simulink model "pstCtrl_testV1"  (R2015a)
settings: Solver=ode45  StartTime=0.0  StopTime=inf  FixedStep=0.05  RelTol=1e-3
values from neighbouring files (symbols this model uses):
  g = 9.81    [PosCntrl_Params.m]
  k_f = m*g/omega_h^2    (= 1.18520816327e-09)    [PosCntrl_Params.m]
  Kdz = 0.4    [PosCntrl_Params.m]
  Kpz = 1.2    [PosCntrl_Params.m]
  m = 0.037    [PosCntrl_Params.m]
  omega_h = 17500    [PosCntrl_Params.m]
  pitch_lb = -40*pi/180    (= -0.698131700798)    [PosCntrl_Params.m]
  pitch_ub = 40*pi/180    (= 0.698131700798)    [PosCntrl_Params.m]
  roll_lb = -40*pi/180    (= -0.698131700798)    [PosCntrl_Params.m]
  roll_ub = 40*pi/180    (= 0.698131700798)    [PosCntrl_Params.m]
  yaw_lb = -pi    (= -3.14159265359)    [PosCntrl_Params.m]
  yaw_ub = pi    (= 3.14159265359)    [PosCntrl_Params.m]
undefined symbols (not defined in the file or in its folder): Kdxx, Kdyy, Kpxy, Kpyx
libraries: aerolibconvert2 x4, CrazyFlie_lib x2, realtime_pacer_lib x2, robotlib x2
settings Model: Creator=rshu  LastModifiedBy=rshu

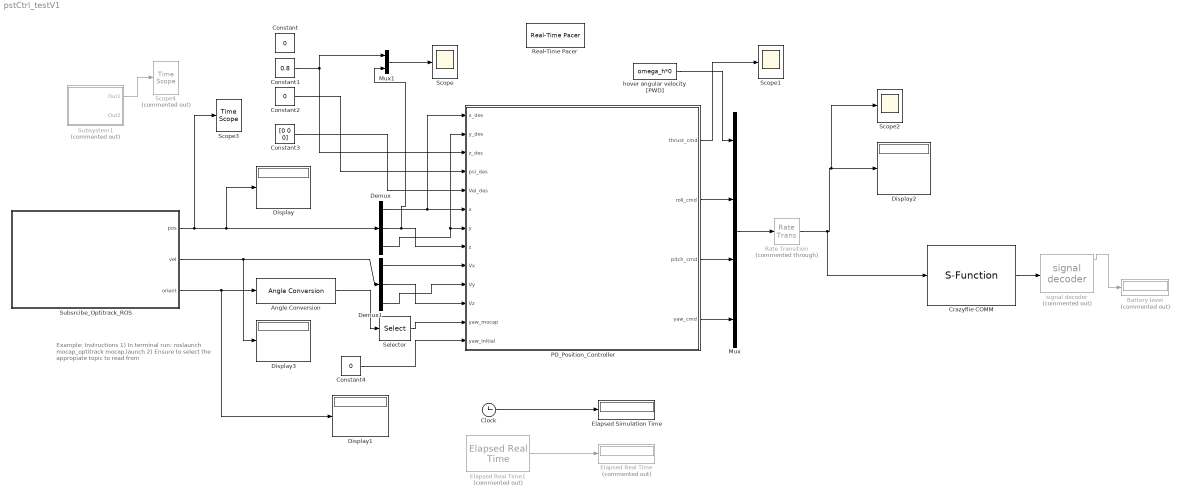
== system pstCtrl_testV1 ==
  note: Example:
      |
      | Instructions
      | 1) In terminal run:
      | roslaunch mocap_optitrack mocap.launch
      | 2) Ensure to select the appropiate topic to read from
  Angle Conversion : aerolibconvert2/Angle Conversion  IU=deg  OU=rad
  Battery level : Display  Commented=on
      settings: Decimation=2
  Clock : Clock
  Constant : Constant  Value=0
  Constant1 : Constant  Value=0.8
  Constant2 : Constant  Value=0
  Constant3 : Constant  Value=[0 0 0]
  Constant4 : Constant  Value=0
  Crazyflie COMM : CrazyFlie_lib/S-Function
  Demux : Demux  Outputs=3
  Demux1 : Demux  Outputs=3
  Display{,1..3} (4 alike) : Display
  Elapsed Real Time : Display  Commented=on
      settings: Decimation=2
  Elapsed Real Time1 : realtime_pacer_lib/Elapsed Real Time  Commented=on
  Elapsed Simulation Time : Display
      settings: Decimation=2
  Mux : Mux
  Mux1 : Mux  Inputs=2
  PD_Position_Controller : Subsystem
  Rate Transition : RateTransition  RequirementInfo="{}  %GIDa_a2c92fb4_87a0_42dd_9129_8c73b2091979"  Commented=through  OutPortSampleTime=sample_time
  Real-Time Pacer : realtime_pacer_lib/Real-Time Pacer  simTimePerRealTime=1
  Scope : Scope
      settings: YMin=0.65  YMax=1
  Scope1 : Scope
      settings: YMin=50468.8  YMax=55781.2
  Scope2 : Scope
      settings: YMin=50468.8  YMax=55781.2  SaveName=ScopeData6
  Scope3 : TimeScope
  Scope4 : TimeScope  Commented=on
  Selector : Selector  InputPortWidth=3  Indices=[2]
  Subsrcibe_Optitrack_ROS : Subsystem
      mask Display:
      | image('prime41-optitrack.png');
      | color('cyan')
      | port_label('output',1,'pos [vector]');
      | port_label('output',2,'vel [vector]');
      | port_label('output',3,'orient [euler]');
  Subsystem1 : Subsystem  Commented=on
  hover angular velocity [PWD] : Constant  Value=omega_h*0
  signal decoder : CrazyFlie_lib/signal decoder  Commented=on
  wires:
  Subsrcibe_Optitrack_ROS/1(pos) -> Demux/1, Display/1, Scope3/1
  Subsrcibe_Optitrack_ROS/2(vel) -> Display3/1, Demux1/1
  Demux/1 -> PD_Position_Controller/1(x_des), PD_Position_Controller/6(x)
  Demux1/1 -> PD_Position_Controller/9(Vx)
  Selector/1 -> PD_Position_Controller/12(yaw_mocap)
  Constant2/1 -> PD_Position_Controller/4(psi_des)
  Constant3/1 -> PD_Position_Controller/5(Vel_des)
  Constant4/1 -> PD_Position_Controller/13(yaw_initial)
  PD_Position_Controller/3(pitch_cmd) -> Mux/3
  PD_Position_Controller/2(roll_cmd) -> Mux/2
  PD_Position_Controller/4(yaw_cmd) -> Mux/4
  Mux/1 -> Rate Transition/1
  Demux/2 -> Mux1/2, PD_Position_Controller/8(z)
  Demux/3 -> PD_Position_Controller/2(y_des), PD_Position_Controller/7(y)
  Demux1/2 -> PD_Position_Controller/11(Vz)
  Demux1/3 -> PD_Position_Controller/10(Vy)
  Constant1/1 -> PD_Position_Controller/3(z_des), Mux1/1
  Subsrcibe_Optitrack_ROS/3(orient) -> Display1/1, Angle Conversion/1
  Angle Conversion/1 -> Selector/1
  Mux1/1 -> Scope/1
  Clock/1 -> Elapsed Simulation Time/1
  Elapsed Real Time1/1 -> Elapsed Real Time/1
  Crazyflie COMM/1 -> signal decoder/1
  signal decoder/1 -> Battery level/1
  PD_Position_Controller/1(thrust_cmd) -> Scope1/1
  hover angular velocity [PWD]/1 -> Mux/1
  Rate Transition/1 -> Crazyflie COMM/1, Scope2/1, Display2/1
  Subsystem1/1(Out1) -> Scope4/1

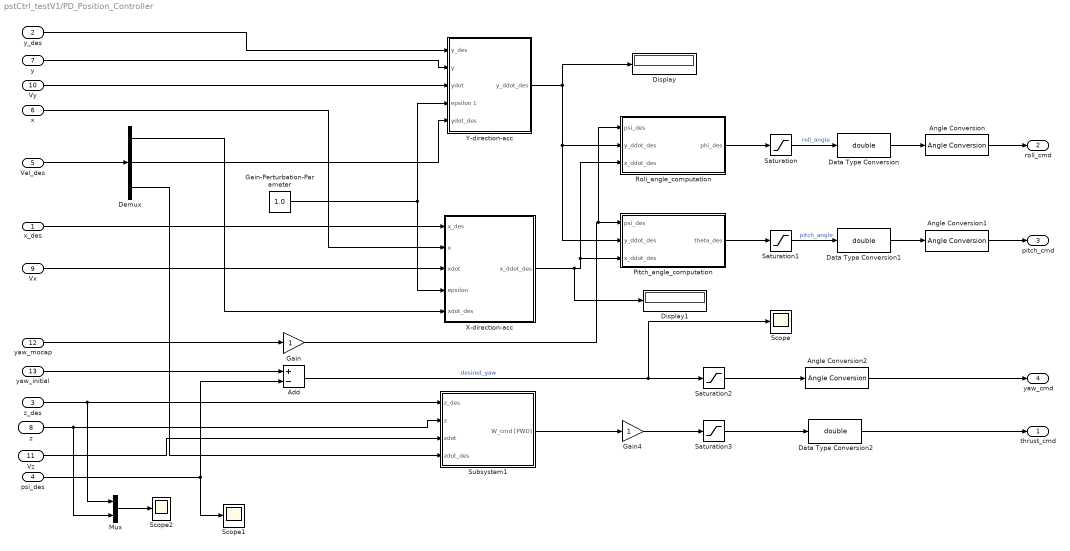
== system pstCtrl_testV1/PD_Position_Controller ==
  x_des : Inport
  y_des : Inport  Port=2
  z_des : Inport  Port=3
  psi_des : Inport  Port=4
  Vel_des : Inport  Port=5
  x : Inport  Port=6
  y : Inport  Port=7
  z : Inport  Port=8
  Vx : Inport  Port=9
  Vy : Inport  Port=10
  Vz : Inport  Port=11
  yaw_mocap : Inport  Port=12
  yaw_initial : Inport  Port=13
  Add : Sum  Inputs=+-
  Angle Conversion : aerolibconvert2/Angle Conversion  IU=rad  OU=deg
  Angle Conversion1 : aerolibconvert2/Angle Conversion  IU=rad  OU=deg
  Angle Conversion2 : aerolibconvert2/Angle Conversion  IU=rad  OU=deg
  Data Type Conversion : DataTypeConversion  OutDataTypeStr=double
  Data Type Conversion1 : DataTypeConversion  OutDataTypeStr=double
  Data Type Conversion2 : DataTypeConversion  OutDataTypeStr=double
  Demux : Demux  Outputs=3
  Display : Display
  Display1 : Display
  Gain : Gain
  Gain-Perturbation-Parameter : Constant  Value=1.0
  Gain4 : Gain
  Mux : Mux  Inputs=2
  Pitch_angle_computation : Subsystem
  Roll_angle_computation : Subsystem
  Saturation : Saturate  UpperLimit=roll_ub  LowerLimit=roll_lb
  Saturation1 : Saturate  UpperLimit=pitch_ub  LowerLimit=pitch_lb
  Saturation2 : Saturate  UpperLimit=yaw_ub  LowerLimit=yaw_lb
  Saturation3 : Saturate  UpperLimit=6e4  LowerLimit=omega_h
  Scope : Scope
      settings: YMin=-1  YMax=1.5  SaveName=ScopeData35
  Scope1 : Scope
      settings: SaveName=ScopeData37
  Scope2 : Scope
      settings: YMin=0.65  YMax=1  SaveName=ScopeData5
  Subsystem1 : Subsystem
  X-direction-acc : Subsystem
  Y-direction-acc : Subsystem
  thrust_cmd : Outport
  roll_cmd : Outport  Port=2
  pitch_cmd : Outport  Port=3
  yaw_cmd : Outport  Port=4
  wires:
  Gain-Perturbation-Parameter/1 -> X-direction-acc/4("epsilon "), Y-direction-acc/4(epsilon 1)
  Roll_angle_computation/1("phi_des ") -> Saturation/1
  Pitch_angle_computation/1("theta_des ") -> Saturation1/1
  X-direction-acc/1(x_ddot_des) -> Display1/1, Roll_angle_computation/3("x_ddot_des "), Pitch_angle_computation/3("x_ddot_des ")
  Y-direction-acc/1(y_ddot_des) -> Roll_angle_computation/2(y_ddot_des), Pitch_angle_computation/2(y_ddot_des), Display/1
  Vy/1 -> Y-direction-acc/3("ydot ")
  Vz/1 -> Subsystem1/3("zdot ")
  y/1 -> Y-direction-acc/2(y)
  Vx/1 -> X-direction-acc/3("xdot ")
  x/1 -> X-direction-acc/2(x)
  Saturation1/1 -> Data Type Conversion1/1  "pitch_angle"
  Saturation/1 -> Data Type Conversion/1  "roll_angle"
  yaw_initial/1 -> Add/1
  Add/1 -> Scope/1, Saturation2/1  "desired_yaw"
  Saturation2/1 -> Angle Conversion2/1
  psi_des/1 -> Scope1/1, Add/2
  z_des/1 -> Mux/1, Subsystem1/1(z_des)
  yaw_mocap/1 -> Gain/1
  Gain/1 -> Roll_angle_computation/1("psi_des "), Pitch_angle_computation/1("psi_des ")
  Gain4/1 -> Saturation3/1
  x_des/1 -> X-direction-acc/1(x_des)
  y_des/1 -> Y-direction-acc/1(y_des)
  Vel_des/1 -> Demux/1
  Demux/2 -> Y-direction-acc/5(ydot_des)
  Demux/1 -> X-direction-acc/5(xdot_des)
  Demux/3 -> Subsystem1/4(zdot_des)
  Data Type Conversion1/1 -> Angle Conversion1/1
  Data Type Conversion2/1 -> thrust_cmd/1
  Data Type Conversion/1 -> Angle Conversion/1
  Angle Conversion/1 -> roll_cmd/1
  Angle Conversion1/1 -> pitch_cmd/1
  Angle Conversion2/1 -> yaw_cmd/1
  Saturation3/1 -> Data Type Conversion2/1
  Subsystem1/1(W_cmd [PWD]) -> Gain4/1
  Mux/1 -> Scope2/1
  z/1 -> Mux/2, Subsystem1/2(z)

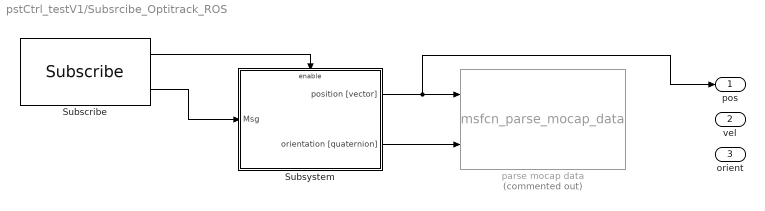
== system pstCtrl_testV1/Subsrcibe_Optitrack_ROS ==
  Subscribe : robotlib/Subscribe  SourceLibraryInfo=This block requires Robotics System Toolbox  topicSource=Select from ROS network  topic=/CF/pose  messageType=geometry_msgs/PoseStamped  sampleTime=-1  messageQueueLength=1
  Subsystem : Subsystem
  parse mocap data : M-S-Function  Commented=on  FunctionName=msfcn_parse_mocap_data
      mask Display:
      | port_label('input', 1, 'pos')
      | port_label('input', 2, 'ornt')
      | 
      | port_label('output', 1, 'pos')
      | port_label('output', 2, 'vel')
      | port_label('output', 3, 'ornt [Euler]')
  pos : Outport
  vel : Outport  Port=2
  orient : Outport  Port=3
  wires:
  Subsystem/1(position [vector]) -> pos/1, parse mocap data/1
  Subscribe/2 -> Subsystem/1(Msg)
  Subscribe/1 -> Subsystem/Enable
  Subsystem/2(orientation [quaternion]) -> parse mocap data/2

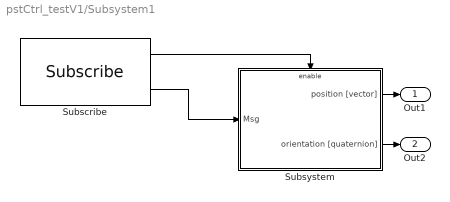
== system pstCtrl_testV1/Subsystem1 ==
  Subscribe : robotlib/Subscribe  SourceLibraryInfo=This block requires Robotics System Toolbox  topicSource=Select from ROS network  topic=/turtle2/pose  messageType=turtlesim/Pose  sampleTime=-1  messageQueueLength=1
  Subsystem : Subsystem
  Out1 : Outport
  Out2 : Outport  Port=2
  wires:
  Subscribe/2 -> Subsystem/1(Msg)
  Subscribe/1 -> Subsystem/Enable
  Subsystem/1(position [vector]) -> Out1/1
  Subsystem/2(orientation [quaternion]) -> Out2/1

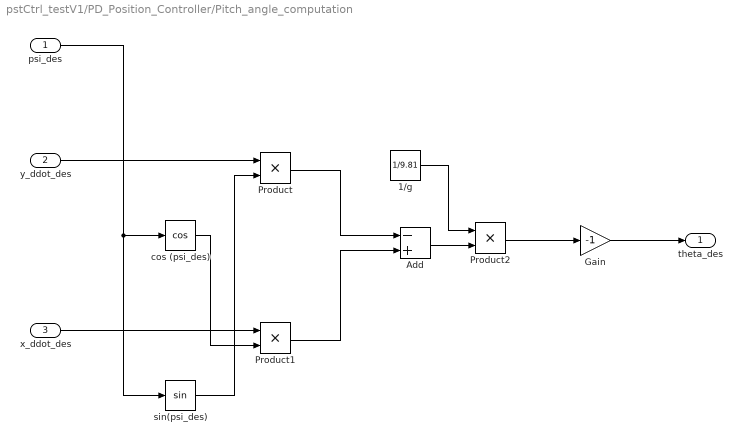
== system pstCtrl_testV1/PD_Position_Controller/Pitch_angle_computation ==
  "psi_des " : Inport
  y_ddot_des : Inport  Port=2
  "x_ddot_des " : Inport  Port=3
  "1/g " : Constant  Value=1/9.81
  Add : Sum  Inputs=-+
  Gain : Gain  Gain=-1
  Product : Product
  Product1 : Product
  Product2 : Product
  cos (psi_des) : Trigonometry  Operator=cos
  sin(psi_des) : Trigonometry
  "theta_des " : Outport
  wires:
  "psi_des "/1 -> cos (psi_des)/1, sin(psi_des)/1
  y_ddot_des/1 -> Product/1
  "x_ddot_des "/1 -> Product1/1
  Product/1 -> Add/1
  Product1/1 -> Add/2
  Add/1 -> Product2/2
  "1/g "/1 -> Product2/1
  Product2/1 -> Gain/1
  Gain/1 -> "theta_des "/1
  cos (psi_des)/1 -> Product1/2
  sin(psi_des)/1 -> Product/2

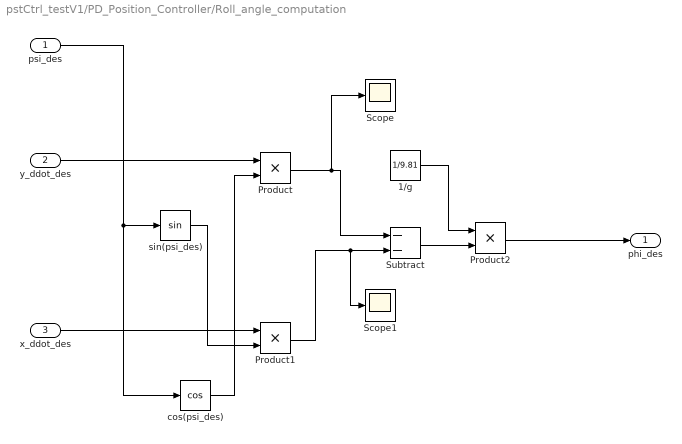
== system pstCtrl_testV1/PD_Position_Controller/Roll_angle_computation ==
  "psi_des " : Inport
  y_ddot_des : Inport  Port=2
  "x_ddot_des " : Inport  Port=3
  "1/g " : Constant  Value=1/9.81
  Product : Product
  Product1 : Product
  Product2 : Product
  Scope : Scope
      settings: TimeRange=30  YMin=-30  YMax=20  SaveName=ScopeData28
  Scope1 : Scope
      settings: TimeRange=30  YMin=-61.5  YMax=-61.3  SaveName=ScopeData30
  Subtract : Sum  Inputs=--
  cos(psi_des) : Trigonometry  Operator=cos
  sin(psi_des) : Trigonometry
  "phi_des " : Outport
  wires:
  "psi_des "/1 -> cos(psi_des)/1, sin(psi_des)/1
  y_ddot_des/1 -> Product/1
  "x_ddot_des "/1 -> Product1/1
  Product/1 -> Scope/1, Subtract/1
  Product1/1 -> Scope1/1, Subtract/2
  Subtract/1 -> Product2/2
  "1/g "/1 -> Product2/1
  Product2/1 -> "phi_des "/1
  sin(psi_des)/1 -> Product1/2
  cos(psi_des)/1 -> Product/2

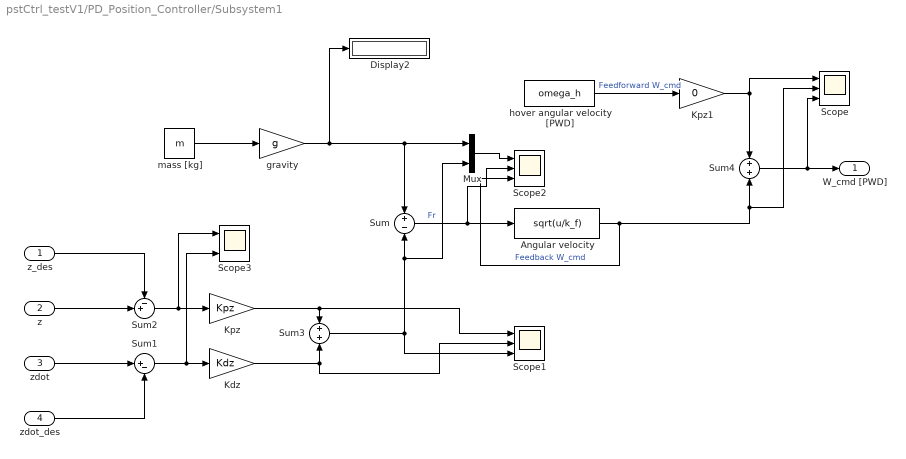
== system pstCtrl_testV1/PD_Position_Controller/Subsystem1 ==
  z_des : Inport
  z : Inport  Port=2
  "zdot " : Inport  Port=3
  zdot_des : Inport  Port=4
  Angular velocity : Fcn  Expr=sqrt(u/k_f)
  Display2 : Display
  Kdz : Gain  Gain=Kdz
  Kpz : Gain  Gain=Kpz
  Kpz1 : Gain  Gain=0
  Mux : Mux  Inputs=2
  Scope : Scope  NumInputPorts=3
      settings: YMin=-5~-5~-5  YMax=5~5~5  SaveName=ScopeData2
  Scope1 : Scope  NumInputPorts=3
      settings: YMin=-5~-5~-5  YMax=5~5~5  SaveName=ScopeData3
  Scope2 : Scope  NumInputPorts=3
      settings: YMin=-0.1~0.2855~38250  YMax=0.4~0.289~38500  SaveName=ScopeData4
  Scope3 : Scope  NumInputPorts=2
      settings: YMin=-0.1~0.2855  YMax=0.4~0.289  SaveName=ScopeData7
  Sum : Sum  Inputs=+|-
  Sum1 : Sum  Inputs=|+-
  Sum2 : Sum  Inputs=-+|
  Sum3 : Sum
  Sum4 : Sum  Inputs=+|+
  gravity : Gain  Gain=g
  hover angular velocity [PWD] : Constant  Value=omega_h
  "mass [kg] " : Constant  Value=m
  W_cmd [PWD] : Outport
  wires:
  "mass [kg] "/1 -> gravity/1
  Sum/1 -> Scope2/2, Angular velocity/1  "Fr"
  "zdot "/1 -> Sum1/1
  zdot_des/1 -> Sum1/2
  Sum1/1 -> Scope3/2, Kdz/1
  z/1 -> Sum2/2
  z_des/1 -> Sum2/1
  Sum2/1 -> Scope3/1, Kpz/1
  Kpz/1 -> Scope1/1, Sum3/1
  Kdz/1 -> Sum3/2, Scope1/2
  Sum3/1 -> Mux/2, Sum/2, Scope1/3
  Angular velocity/1 -> Scope2/3, Scope/2, Sum4/2  "Feedback W_cmd"
  Sum4/1 -> Scope/3, W_cmd [PWD]/1
  hover angular velocity [PWD]/1 -> Kpz1/1  "Feedforward W_cmd"
  gravity/1 -> Display2/1, Mux/1, Sum/1
  Kpz1/1 -> Sum4/1, Scope/1
  Mux/1 -> Scope2/1

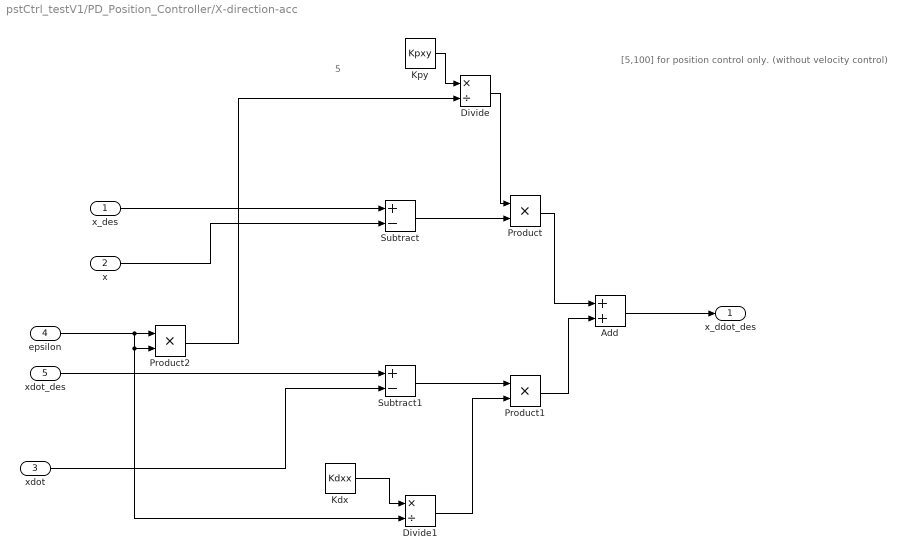
== system pstCtrl_testV1/PD_Position_Controller/X-direction-acc ==
  note: [5,100] for position control only. (without velocity control)
  note: 5
  x_des : Inport
  x : Inport  Port=2
  "xdot " : Inport  Port=3
  "epsilon " : Inport  Port=4
  xdot_des : Inport  Port=5
  Add : Sum
  Divide : Product  Inputs=*/
  Divide1 : Product  Inputs=*/
  "Kdx " : Constant  Value=Kdxx
  Kpy : Constant  Value=Kpxy
  Product : Product
  Product1 : Product
  Product2 : Product
  Subtract : Sum  Inputs=+-
  Subtract1 : Sum  Inputs=+-
  x_ddot_des : Outport
  wires:
  x/1 -> Subtract/2
  x_des/1 -> Subtract/1
  Subtract/1 -> Product/2
  Subtract1/1 -> Product1/1
  Product1/1 -> Add/2
  Product/1 -> Add/1
  Add/1 -> x_ddot_des/1
  "xdot "/1 -> Subtract1/2
  Divide/1 -> Product/1
  Kpy/1 -> Divide/1
  "Kdx "/1 -> Divide1/1
  Divide1/1 -> Product1/2
  "epsilon "/1 -> Divide1/2, Product2/2, Product2/1
  Product2/1 -> Divide/2
  xdot_des/1 -> Subtract1/1

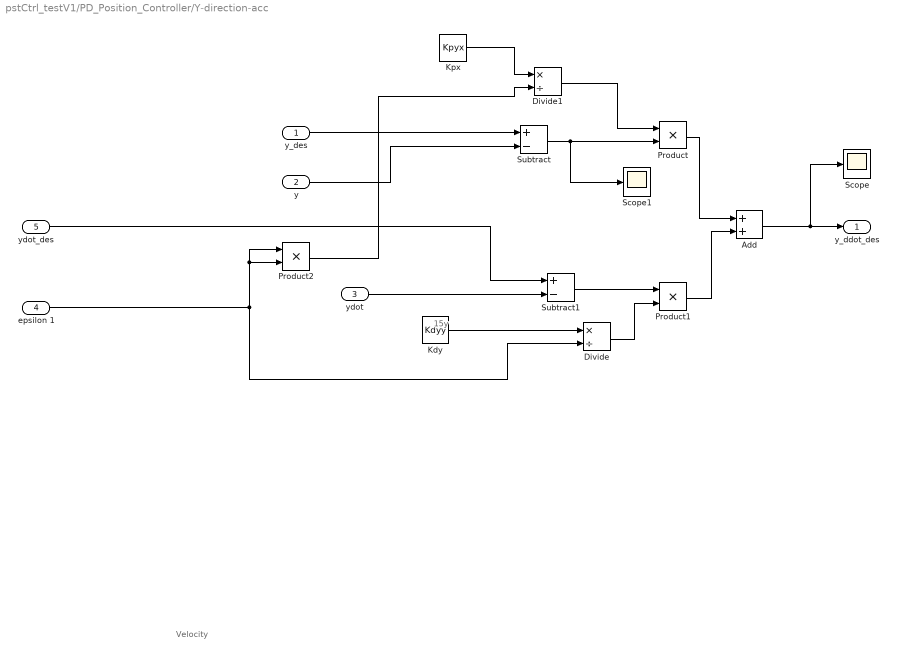
== system pstCtrl_testV1/PD_Position_Controller/Y-direction-acc ==
  note: Velocity
  note: 15y
  y_des : Inport
  y : Inport  Port=2
  "ydot " : Inport  Port=3
  epsilon 1 : Inport  Port=4
  ydot_des : Inport  Port=5
  Add : Sum
  Divide : Product  Inputs=*/
  Divide1 : Product  Inputs=*/
  "Kdy " : Constant  Value=Kdyy
  Kpx : Constant  Value=Kpyx
  Product : Product
  Product1 : Product
  Product2 : Product
  Scope : Scope
      settings: TimeRange=50  YMin=-4.5  YMax=-1.5  SaveName=ScopeData29
  Scope1 : Scope
      settings: TimeRange=50  YMin=-2  YMax=2  SaveName=ScopeData21
  Subtract : Sum  Inputs=+-
  Subtract1 : Sum  Inputs=+-
  y_ddot_des : Outport
  wires:
  y/1 -> Subtract/2
  "ydot "/1 -> Subtract1/2
  y_des/1 -> Subtract/1
  Subtract/1 -> Scope1/1, Product/2
  Subtract1/1 -> Product1/1
  Product1/1 -> Add/2
  Product/1 -> Add/1
  Add/1 -> Scope/1, y_ddot_des/1
  epsilon 1/1 -> Divide/2, Product2/2, Product2/1
  Product2/1 -> Divide1/2
  Kpx/1 -> Divide1/1
  "Kdy "/1 -> Divide/1
  Divide/1 -> Product1/2
  Divide1/1 -> Product/1
  ydot_des/1 -> Subtract1/1

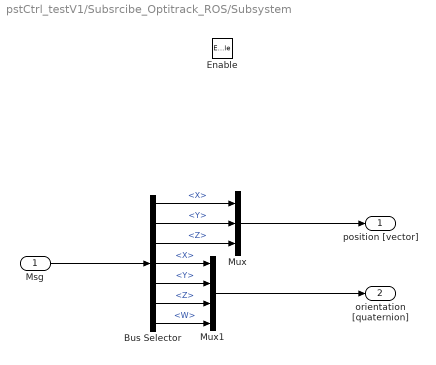
== system pstCtrl_testV1/Subsrcibe_Optitrack_ROS/Subsystem ==
  Msg : Inport
  Enable : EnablePort
  Bus Selector : BusSelector  OutputSignals=Pose.Position.X,Pose.Position.Y,Pose.Position.Z,Pose.Orientation.X,Pose.Orientation.Y,Pose.Orientation.Z,Pose.Orientation.W
  Mux : Mux  Inputs=3
  Mux1 : Mux
  position [vector] : Outport
  orientation [quaternion] : Outport  Port=2
  wires:
  Msg/1 -> Bus Selector/1
  Bus Selector/1 -> Mux/1  "<X>"
  Bus Selector/2 -> Mux/2  "<Y>"
  Bus Selector/3 -> Mux/3  "<Z>"
  Mux/1 -> position [vector]/1
  Bus Selector/4 -> Mux1/1  "<X>"
  Bus Selector/5 -> Mux1/2  "<Y>"
  Bus Selector/6 -> Mux1/3  "<Z>"
  Bus Selector/7 -> Mux1/4  "<W>"
  Mux1/1 -> orientation [quaternion]/1

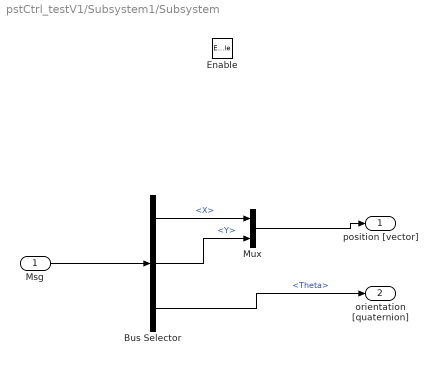
== system pstCtrl_testV1/Subsystem1/Subsystem ==
  Msg : Inport
  Enable : EnablePort
  Bus Selector : BusSelector  OutputSignals=X,Y,Theta
  Mux : Mux  Inputs=2
  position [vector] : Outport
  orientation [quaternion] : Outport  Port=2
  wires:
  Msg/1 -> Bus Selector/1
  Bus Selector/1 -> Mux/1  "<X>"
  Bus Selector/2 -> Mux/2  "<Y>"
  Mux/1 -> position [vector]/1
  Bus Selector/3 -> orientation [quaternion]/1  "<Theta>"
